simulink subsystem "Sensors"  (R2025a)
settings: Solver=VariableStepAuto  StartTime=0.0  StopTime=10.0  RelTol=1e-3
undefined symbols (not defined in the file): config, DiscIntNeverNeededParam
settings Model: Creator=Jackt  LastModifiedBy=Jackt

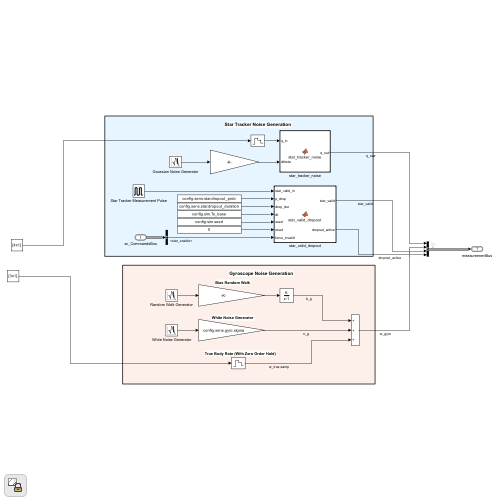
[thumbnail: Simulink's stored preview of the top-level diagram]
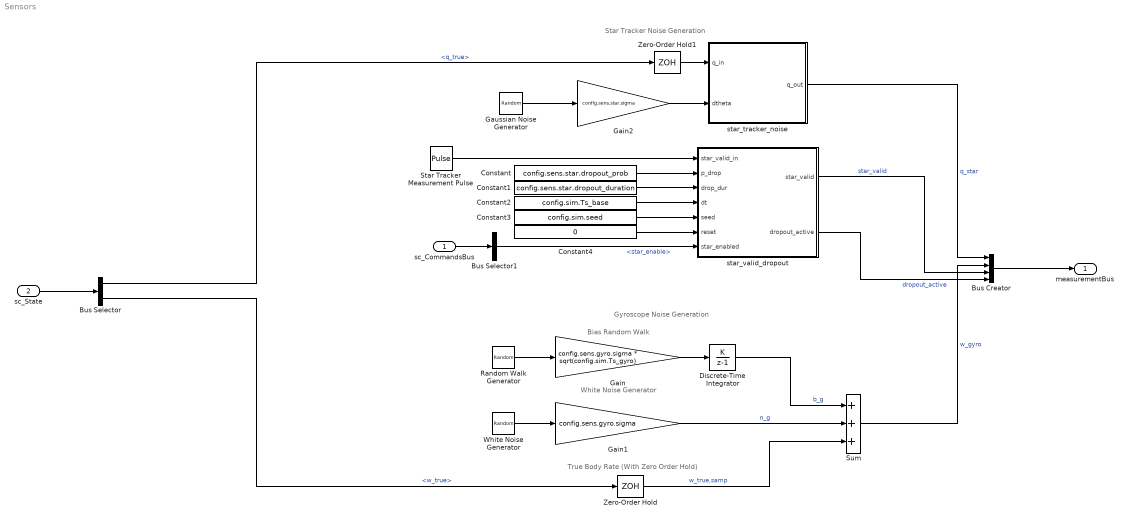
== system Sensors ==
  note: Gyroscope Noise Generation
  note: True Body Rate (With Zero Order Hold)
  note: White Noise Generator
  note: Bias Random Walk
  note: Star Tracker Noise Generation
  sc_CommandsBus : Inport  OutDataTypeStr=Bus: commandBus
  sc_State : Inport  Port=2  OutDataTypeStr=Bus: sc_stateBus
  Bus Creator : BusCreator  Inputs=4  OutDataTypeStr=Bus: measurementBus
  Bus Selector : BusSelector  OutputSignals=q_true,w_true
  Bus Selector1 : BusSelector  OutputSignals=star_enable
  Constant : Constant  Value=config.sens.star.dropout_prob  VectorParams1D=off
  Constant1 : Constant  Value=config.sens.star.dropout_duration  VectorParams1D=off
  Constant2 : Constant  Value=config.sim.Ts_base  VectorParams1D=off
  Constant3 : Constant  Value=config.sim.seed  VectorParams1D=off
  Constant4 : Constant  Value=0
  Discrete-Time Integrator : DiscreteIntegrator  IntegratorMethod=Accumulation: Forward Euler  InitialCondition=config.est.bias_0  SampleTime=config.sim.Ts_gyro  ICPrevOutput=DiscIntNeverNeededParam  ICPrevScaledInput=DiscIntNeverNeededParam
  Gain : Gain  Gain=config.sens.gyro.sigma * sqrt(config.sim.Ts_gyro)
  Gain1 : Gain  Gain=config.sens.gyro.sigma
  Gain2 : Gain  Gain=config.sens.star.sigma
  Gaussian Noise Generator : RandomNumber  Mean=[0; 0; 0]  Variance=[1; 1; 1]  Seed=config.sim.seed  SampleTime=config.sim.Ts_star  VectorParams1D=off
  Random Walk Generator : RandomNumber  Mean=[0; 0; 0]  Variance=[1; 1; 1]  Seed=config.sim.seed  SampleTime=config.sim.Ts_gyro  VectorParams1D=off
  Star Tracker Measurement Pulse : DiscretePulseGenerator  PulseType=Time based  Period=config.sim.Ts_star  PulseWidth=100*config.sim.Ts_base/config.sim.Ts_star  VectorParams1D=off
  Sum : Sum  Inputs=+++
  White Noise Generator : RandomNumber  Mean=[0; 0; 0]  Variance=[1; 1; 1]  Seed=config.sim.seed  SampleTime=config.sim.Ts_gyro  VectorParams1D=off
  Zero-Order Hold : ZeroOrderHold  SampleTime=config.sim.Ts_gyro
  Zero-Order Hold1 : ZeroOrderHold  SampleTime=config.sim.Ts_star
  star_tracker_noise : MATLAB Function  TreatAsAtomicUnit=on
  star_valid_dropout : MATLAB Function  TreatAsAtomicUnit=on
  measurementBus : Outport  OutDataTypeStr=Bus: measurementBus
  wires:
  Bus Selector/1 -> Zero-Order Hold1/1  "<q_true>"
  Bus Selector/2 -> Zero-Order Hold/1  "<w_true>"
  Random Walk Generator/1 -> Gain/1
  Gain/1 -> Discrete-Time Integrator/1
  Discrete-Time Integrator/1 -> Sum/1  "b_g"
  White Noise Generator/1 -> Gain1/1
  Gain1/1 -> Sum/2  "n_g"
  Zero-Order Hold/1 -> Sum/3  "w_true,samp"
  Sum/1 -> Bus Creator/2  "w_gyro"
  Gaussian Noise Generator/1 -> Gain2/1
  Zero-Order Hold1/1 -> star_tracker_noise/1(q_in)
  Gain2/1 -> star_tracker_noise/2(dtheta)
  star_tracker_noise/1(q_out) -> Bus Creator/1  "q_star"
  Star Tracker Measurement Pulse/1 -> star_valid_dropout/1(star_valid_in)
  star_valid_dropout/1(star_valid) -> Bus Creator/3  "star_valid"
  Constant/1 -> star_valid_dropout/2(p_drop)
  Constant1/1 -> star_valid_dropout/3(drop_dur)
  Constant3/1 -> star_valid_dropout/5(seed)
  Constant4/1 -> star_valid_dropout/6(reset)
  star_valid_dropout/2(dropout_active) -> Bus Creator/4  "dropout_active"
  Constant2/1 -> star_valid_dropout/4(dt)
  Bus Selector1/1 -> star_valid_dropout/7(star_enabled)  "<star_enable>"
  sc_CommandsBus/1 -> Bus Selector1/1
  Bus Creator/1 -> measurementBus/1
  sc_State/1 -> Bus Selector/1

== matlab function Sensors/star_tracker_noise ==
  data: q_in input; q_out output; dtheta input
function q_out = star_tracker_noise(q_in, dtheta)
%STAR_TRACKER_NOISE Apply star-tracker attitude noise to a quaternion.

%Enforce Shapes
q = q_in(:);
d = dtheta(:);

%Input Check
if numel(q) ~= 4 || numel(d) ~= 3 || any(~isfinite(q)) || any(~isfinite(d))
    q_out = [1;0;0;0];
    return;
end

%Normalize Input Quaternions
nq = norm(q);
if nq < 1e-12
    q = [1;0;0;0];
else
    q = q / nq;
end

%Map rotation vector noise to quaternion via exponential map
theta = norm(d);

if theta < 1e-12
    dq = [1;0;0;0];
else
    u = d / theta; %unit axis
    half = 0.5 * theta;
    dq = [cos(half); u * sin(half)];
end

%Measured attitude = true attitude * noise
q_out = quatmultiply_sf(q, dq);

%Normalize output
no = norm(q_out);
if no < 1e-12
    q_out = [1;0;0;0];
else
    q_out = q_out / no;
end

%Format for Simulink Processing
q_out = reshape(q_out, [4 1]);

end


function q = quatmultiply_sf(a,b)
%QUATMULTIPLY_SF Scalar-first quaternion multiply: q = a ⊗ b
% a,b,q are [4x1] with scalar first.
w1=a(1); x1=a(2); y1=a(3); z1=a(4);
w2=b(1); x2=b(2); y2=b(3); z2=b(4);

q = [ w1*w2 - x1*x2 - y1*y2 - z1*z2;
      w1*x2 + x1*w2 + y1*z2 - z1*y2;
      w1*y2 - x1*z2 + y1*w2 + z1*x2;
      w1*z2 + x1*y2 - y1*x2 + z1*w2 ];
end

== matlab function Sensors/star_valid_dropout ==
  settings: updateMethod=DISCRETE
  data: star_valid_in input; p_drop input; drop_dur input; dt input; seed input; star_valid output; dropout_active output; reset input; star_enabled input
function [star_valid, dropout_active] = star_valid_dropout(star_valid_in, p_drop, drop_dur, dt, seed, reset, star_enabled)
%Star tracker validity with probabilistic dropout and fixed duration

%Track variables across iterations of this function
persistent is_init active count target

%Flip Startracker force-invalid from star-tracker-enabled
force_invalid = ~star_enabled;

%If this is the first run of this function, initialize variables
if isempty(is_init) || reset
    is_init = true;
    active = false;
    count = int32(0);
    target = int32(0);
    rng(seed, "twister");
end

%Clamp inputs
if p_drop < 0, p_drop = 0; end
if p_drop > 1, p_drop = 1; end
if drop_dur < 0, drop_dur = 0; end
if dt <= 0, dt = 1; end

%If dropout not active, decide whether to start one
if ~active
    u = rand();
    if u < p_drop
        active = true;
        count = int32(0);
        target = int32(ceil(drop_dur / dt));
        if target < 1
            target = int32(1);
        end
        star_valid = 0;
        dropout_active = 1;
    else
        star_valid = star_valid_in;
        dropout_active = 0;
    end

%If dropout active, block output and advance counter
else
    star_valid = 0;
    dropout_active = 1;

    count = count + 1;
    if count >= target
        active = false;
        count = int32(0);
        target = int32(0);
        star_valid = star_valid_in;
        dropout_active = 0;
    end
end

if(force_invalid)
    star_valid = 0;
end

%Format shape for Simulink
star_valid = double(star_valid(1));
dropout_active = double(dropout_active(1));

end
